simulink model "FW_formation_control_wind"  (R2023b)
settings: Solver=FixedStepAuto  StartTime=0.0  StopTime=70  FixedStep=0.001  RelTol=1e-3
undefined symbols (not defined in the file or in its folder): C, com, fc, hc, init, L, L2, lc, leader, tau, Va_max, Va_min
libraries: Fixed_Wing x3, simulink x1
(part 1 of 2)
settings Model: Creator=TigerWuu  LastModifiedBy=NCS
settings SolverCC: MaxConsecutiveMinStep=10  ZeroCrossAlgorithm=Adaptive  EnableFixedStepZeroCrossing=on
settings OptimizationCC: EnhancedBackFolding=on  PassReuseOutputArgsAs=Individual arguments  ZeroExternalMemoryAtStartup=off  ZeroInternalMemoryAtStartup=off  MaxStackSize=64  OptimizeBlockOrder=speed  DifferentSizesBufferReuse=on  OptimizationCustomize=off  EfficientTunableParamExpr=on
settings DebuggingCC: IgnoredZcDiagnostic=none  ParameterTunabilityLossMsg=error  UnconnectedInputMsg=warning  UnconnectedOutputMsg=warning  UnconnectedLineMsg=warning  UnderSpecifiedDimensionMsg=warning
settings HardwareCC: UseEmbeddedCoderFeatures=off
settings ModelReferenceCC: EnableRefExpFcnMdlSchedulingChecks=on
settings SFSimCC: MATLABDynamicMemAlloc=off
settings RTWCC: Description=Embedded Coder  SystemTargetFile=ert.tlc  HardwareBoard=Robot Operating System 2 (ROS 2)  TLCOptions="-aInlineSetEventsForThisBaseRateFcn=TLC_FALSE -aSuppressMultiTaskScheduler=TLC_FALSE  -aRateBasedStepFcn=0"  TemplateMakefile=ert_default_tmf  Toolchain=Colcon Tools  TargetLang=C++  DLArmComputeVersion=19.05
settings CodeAppCC: ForceParamTrailComments=on  IgnoreCustomStorageClasses=off  OperatorAnnotations=on  SimulinkDataObjDesc=on  SFDataObjDesc=on  InsertBlockDesc=on
settings ERTTargetCC: CodeInterfacePackaging=C++ class  SupportNonInlinedSFcns=on  RootIOFormat=Structure reference

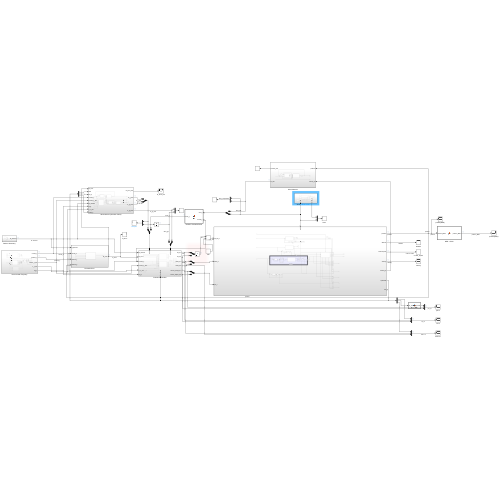
[thumbnail: Simulink's stored preview of the top-level diagram]
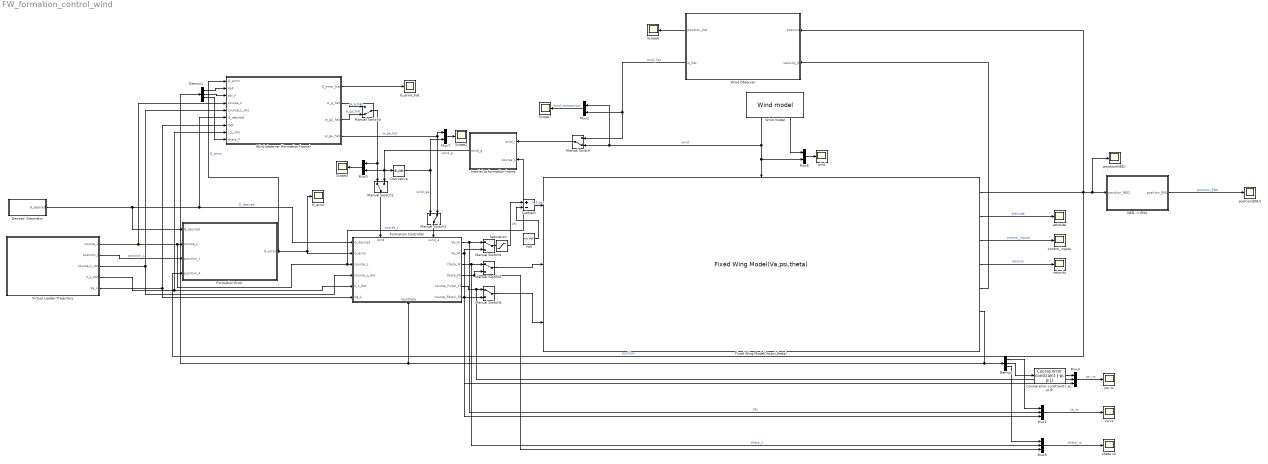
== system FW_formation_control_wind ==
  "Course error constraint [-pi, pi]1" : Fixed_Wing/Fixed Wing Model(Va,psi,theta)/Course error constraint [-pi, pi]1  SystemSampleTime=-1  VariantActivationTime=update diagram  AllowFlexibleInterface=on  Latency=0  AutoFrameSizeCalculation=off
      settings: SourceProductName=Fixed-Wing Model
  Demux : Demux  Outputs=3
  Demux1 : Demux  Outputs=3
  Derivative : Derivative
  Desired  Geometry : Subsystem
  Fixed Wing Model(Va,psi,theta) : Fixed_Wing/Fixed Wing Model(Va,psi,theta)  SystemSampleTime=-1  VariantActivationTime=update diagram  AllowFlexibleInterface=on  Latency=0  AutoFrameSizeCalculation=off
      link override Integrator: InitialCondition=init.psi0
      link override Integrator2: InitialCondition=init.psi0
      link override Ki_course: Gain=0
      settings: SourceProductName=Fixed-Wing Model  PortSchema="{\"entries\":[{\"content\":{\"sides\":[{\"content\":{\"connectorIds\":[\"In1\",\"In2\",\"In3\"]},\"type\":\"ConnectorPlacement.EquallySpacedRectSide\",\"uuid\":\"491080cc-ba33-4dca-9b37-922a1b131a7c\"},{\"content\":{\"connectorIds\":[\"Out1\",\"Out2\",\"Out3\",\"Out4\",\"Out5\",\"Out6\",\"Out7\"],\"side\":\"RIGHT\"},\"type\":\"ConnectorPlacement.EquallySpacedRectSide\",\"uuid\":\"e4e8ca81-264a-41b3-9d62-a2cb565f7b79\"},{\"content\":{\"connectorIds\":[\"In4\"],\"side\":\"TOP\"},\"type\":\"ConnectorPlacement.EquallySpacedRectSide\",\"uuid\":\"52444ebc-de17-4d3c-95e2-2270054ae63e\"},{\"content\":{\"side\":\"BOTTOM\"},\"type\":\"ConnectorPlacement.EquallySpacedRectSide\",\"uuid\":\"cd38afea-0687-422f-bcb3-a9854084c98f\"}]},\"type\":\"ConnectorPlacement.EquallySpacedConnector\",\"uuid\":\"020d1068-73e8-421c-b651-66bcdf43a07b\"}],\"packageUris\":[\"http://schema.mathworks.com/mf0/Connector/R2020b\"],\"version\":\"1.0\"}"
  Formation Controller : Subsystem
      settings: PortSchema="{\"entries\":[{\"content\":{\"sides\":[{\"content\":{\"connectorIds\":[\"In1\",\"In2\",\"In3\",\"In4\",\"In5\",\"In6\"]},\"type\":\"ConnectorPlacement.EquallySpacedRectSide\",\"uuid\":\"9c389f85-23f7-4ad0-9870-58a1e0934639\"},{\"content\":{\"connectorIds\":[\"Out1\",\"Out2\",\"Out3\",\"Out4\",\"Out5\",\"Out6\"],\"side\":\"RIGHT\"},\"type\":\"ConnectorPlacement.EquallySpacedRectSide\",\"uuid\":\"ce3247c4-1bae-44d3-b9da-13662f8788fa\"},{\"content\":{\"connectorIds\":[\"In7\",\"In8\"],\"side\":\"TOP\"},\"type\":\"ConnectorPlacement.EquallySpacedRectSide\",\"uuid\":\"1a627aed-9846-48b6-b280-b2fda66f57fb\"},{\"content\":{\"connectorIds\":[\"In9\"],\"side\":\"BOTTOM\"},\"type\":\"ConnectorPlacement.EquallySpacedRectSide\",\"uuid\":\"66985a5e-001d-400a-88a5-7872307471ad\"}]},\"type\":\"ConnectorPlacement.EquallySpacedConnector\",\"uuid\":\"4ccca4c3-7c97-47a5-8a1e-b96349422d36\"}],\"packageUris\":[\"http://schema.mathworks.com/mf0/Connector/R2020b\"],\"version\":\"1.0\"}"
  Formation Error : Subsystem
  G_error : Scope
  G_error_hat : Scope
  Inertial to formation frame : MATLAB Function  TreatAsAtomicUnit=on
  Manual Switch : ManualSwitch  CurrentSetting=0
  Manual Switch{1,4..6} (4 alike) : ManualSwitch
  Manual Switch2 : ManualSwitch  CurrentSetting=0
  Manual Switch3 : ManualSwitch  CurrentSetting=0
  Mux1 : Mux  Inputs=3
  Mux{2..3,6..7} (4 alike) : Mux  Inputs=2
  Mux4 : Mux  Inputs=3
  Mux5 : Mux  Inputs=3
  "NED -> ENU" : MATLAB Function  TreatAsAtomicUnit=on
  Saturation : Saturate  UpperLimit=Va_max  LowerLimit=Va_min
  Scope{2..3,6..7} (4 alike) : Scope
  Subtract : Sum  Inputs=+-
  Va0 : Constant  Value=init.Va0
  Virtual Leader Trajectory : Subsystem
  Wind Observer : Subsystem
  Wind model : Fixed_Wing/Wind model  SystemSampleTime=-1  VariantActivationTime=update diagram  AllowFlexibleInterface=on  Latency=0  AutoFrameSizeCalculation=off
      link override Steady wind /Gain: Gain=1
      link override Steady wind /Gain1: Gain=-2
      link override Steady wind /wd: Value=0
      link override Steady wind gust/Gain: Gain=0.2
      link override Steady wind gust/Gain1: Gain=0.2
      link override Steady wind gust/Gain2: Gain=1
      link override Steady wind gust/Gain3: Gain=-1
      link override Steady wind gust/Gain4: Gain=0.7
      settings: SourceProductName=Fixed-Wing Model  PortSchema="{\"entries\":[{\"content\":{\"sides\":[{\"content\":{},\"type\":\"ConnectorPlacement.EquallySpacedRectSide\",\"uuid\":\"19ef0eb7-c626-45ec-b76b-8668fc024824\"},{\"content\":{\"side\":\"RIGHT\"},\"type\":\"ConnectorPlacement.EquallySpacedRectSide\",\"uuid\":\"89e72569-ab94-4162-a6e2-b425ef08f724\"},{\"content\":{\"side\":\"TOP\"},\"type\":\"ConnectorPlacement.EquallySpacedRectSide\",\"uuid\":\"6d9409e9-6822-4cd9-902f-e5665cb68433\"},{\"content\":{\"connectorIds\":[\"Out1\",\"Out2\"],\"side\":\"BOTTOM\"},\"type\":\"ConnectorPlacement.EquallySpacedRectSide\",\"uuid\":\"39a83352-0924-44fa-be5d-94a7c28bbbf3\"}]},\"type\":\"ConnectorPlacement.EquallySpacedConnector\",\"uuid\":\"6cf6ae00-ef23-42a2-99b2-ca60e191fb03\"}],\"packageUris\":[\"http://schema.mathworks.com/mf0/Connector/R2020b\"],\"version\":\"1.0\"}"
  Wind observer (formation frame) : Subsystem
  attitude : Scope
  control_inputs : Scope
  position(ENU) : Scope
  position(NED) : Scope
  psi vs : Scope
  theta vs : Scope
  va vs : Scope
  velocity : Scope
  wind : Scope
  wires:
  Fixed Wing Model(Va,psi,theta)/1 -> position(NED)/1, "NED -> ENU"/1(position_NED), Formation Error/4(position_F), Wind Observer/1(position)  "position"
  Fixed Wing Model(Va,psi,theta)/3 -> control_inputs/1  "control_inputs"
  "NED -> ENU"/1(position_ENU) -> position(ENU)/1  "position_ENU"
  Virtual Leader Trajectory/2(position_L) -> Formation Error/3(position_L)  "position_L"
  Virtual Leader Trajectory/1(course_L) -> Wind observer (formation frame)/4(course_L), Inertial to formation frame/2(course_L), Formation Controller/3(course_L), Formation Error/2(course_L)  "course_L"
  Desired  Geometry/1(G_desired) -> Formation Error/1(G_desired), Wind observer (formation frame)/6(G_desired), Formation Controller/1(G_desired)  "G_desired"
  Virtual Leader Trajectory/3(course_L_dot) -> Formation Controller/4(course_L_dot), Wind observer (formation frame)/5(course_L_dot)
  Virtual Leader Trajectory/5(Vg_L) -> Formation Controller/6(Vg_L), Wind observer (formation frame)/7(VgL)
  Formation Error/1(G_error) -> Wind observer (formation frame)/1(G_error), G_error/1, Formation Controller/2(G_error)  "G_error"
  Wind model/1 -> Fixed Wing Model(Va,psi,theta)/4, Mux6/2, Mux2/1, Manual Switch/2  "wind"
  Formation Controller/5(course_Fc/psi_Fc) -> Mux4/2, Manual Switch6/1
  Fixed Wing Model(Va,psi,theta)/2 -> attitude/1  "attitude"
  Fixed Wing Model(Va,psi,theta)/4 -> velocity/1  "velocity"
  Subtract/1 -> Fixed Wing Model(Va,psi,theta)/1  "V_F_bar"
  Va0/1 -> Subtract/2
  Fixed Wing Model(Va,psi,theta)/5 -> Wind Observer/2(velocity_0)
  Wind Observer/1(position_hat) -> Scope6/1
  Mux2/1 -> Scope7/1  "wind_comparison"
  Wind Observer/2(w_hat) -> Manual Switch/1, Mux2/2  "wind_hat"
  Demux1/2 -> Wind observer (formation frame)/3(psi_F)
  Demux1/1 -> Wind observer (formation frame)/2(VaF)
  Fixed Wing Model(Va,psi,theta)/6 -> Demux/1, Demux1/1, Formation Controller/9(Vpsitheta)
  Wind observer (formation frame)/1(G_error_hat) -> G_error_hat/1
  Manual Switch/1 -> Inertial to formation frame/1(wind_i)
  Manual Switch1/1 -> Formation Controller/7(wind)
  Inertial to formation frame/1(wind_g) -> Mux3/2, Derivative/1, Manual Switch1/2  "wind_g"
  Mux3/1 -> Scope3/1
  Virtual Leader Trajectory/4(z_L_dot) -> Formation Controller/5(z_L_dot), Wind observer (formation frame)/8(z_L_dot)
  Saturation/1 -> Subtract/1  "VFc"
  Mux1/1 -> va vs/1  "va_vs"
  Mux4/1 -> psi vs/1  "psi_vs"
  Formation Controller/3(theta_Fc) -> Manual Switch5/1, Mux5/2  "theta_c"
  Mux5/1 -> theta vs/1  "theta_vs"
  Formation Controller/6(course_Fd/psi_Fd) -> Manual Switch6/2, Mux4/3
  Formation Controller/2(Va_Fd) -> Manual Switch4/2, Mux1/3
  Mux6/1 -> wind/1
  Wind model/2 -> Mux6/1
  Derivative/1 -> Manual Switch2/1, Mux7/2  "wind_ga"
  Mux7/1 -> Scope2/1
  Wind observer (formation frame)/4(w_ga_hat) -> Mux7/1, Manual Switch2/2  "w_ga_hat"
  Manual Switch2/1 -> Formation Controller/8(wind_a)
  Formation Controller/4(theta_Fd) -> Mux5/3, Manual Switch5/2
  Demux1/3 -> Wind observer (formation frame)/9(theta_F)
  Demux/1 -> Mux1/1
  Demux/2 -> "Course error constraint [-pi, pi]1"/1
  Demux/3 -> Mux5/1
  Wind observer (formation frame)/3(w_g2_hat) -> Manual Switch3/2  "w_g2_hat"
  Wind observer (formation frame)/2(w_g_hat) -> Manual Switch3/1  "w_g_hat"
  Manual Switch3/1 -> Manual Switch1/1, Mux3/1
  "Course error constraint [-pi, pi]1"/1 -> Mux4/1
  Formation Controller/1(Va_Fc) -> Mux1/2, Manual Switch4/1  "VFc"
  Manual Switch4/1 -> Saturation/1
  Manual Switch5/1 -> Fixed Wing Model(Va,psi,theta)/2
  Manual Switch6/1 -> Fixed Wing Model(Va,psi,theta)/3

== system FW_formation_control_wind/Desired  Geometry ==
  Mux : Mux  Inputs=3
  fc : Constant  Value=fc(2)
  hc : Constant  Value=hc(2)
  lc : Constant  Value=lc(2)
  G_desired : Outport
  wires:
  Mux/1 -> G_desired/1  "desired geometry"
  lc/1 -> Mux/1
  fc/1 -> Mux/2
  hc/1 -> Mux/3

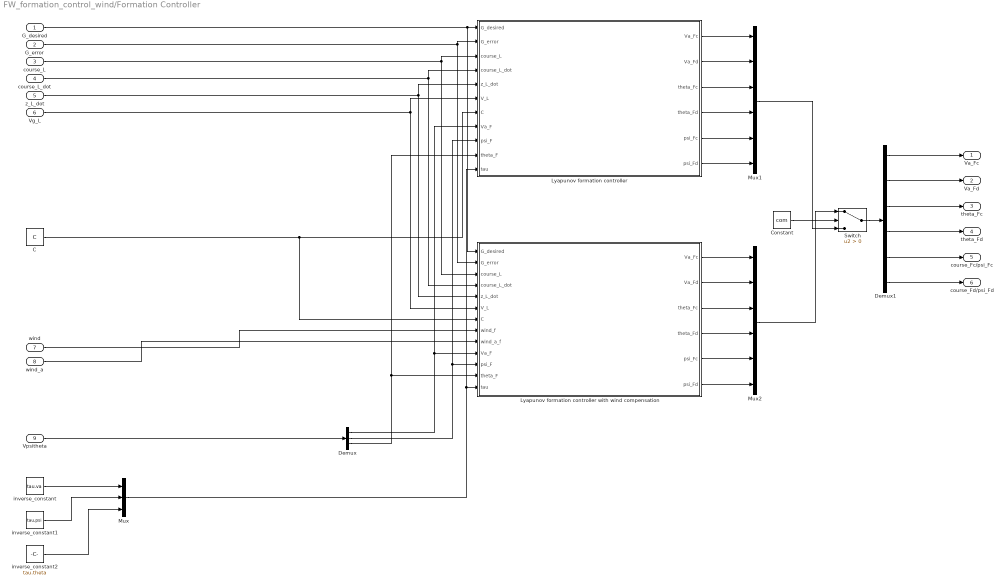
== system FW_formation_control_wind/Formation Controller ==
  G_desired : Inport
  G_error : Inport  Port=2
  course_L : Inport  Port=3
  course_L_dot : Inport  Port=4
  z_L_dot : Inport  Port=5
  Vg_L : Inport  Port=6
  wind : Inport  Port=7
  wind_a : Inport  Port=8
  Vpsitheta : Inport  Port=9
  C : Constant  Value=C
  Constant : Constant  Value=com
  Demux : Demux  Outputs=3
  Demux1 : Demux  Outputs=6
  Lyapunov formation controller : MATLAB Function  TreatAsAtomicUnit=on
  Lyapunov formation controller with wind compensation : MATLAB Function  TreatAsAtomicUnit=on
  Mux : Mux  Inputs=3
  Mux1 : Mux  Inputs=6
  Mux2 : Mux  Inputs=6
  Switch : Switch  Criteria=u2 > Threshold  SaturateOnIntegerOverflow=off  InputSameDT=off
  inverse_constant : Constant  Value=tau.va
  inverse_constant1 : Constant  Value=tau.psi
  inverse_constant2 : Constant  Value=tau.theta
  Va_Fc : Outport
  Va_Fd : Outport  Port=2
  theta_Fc : Outport  Port=3
  theta_Fd : Outport  Port=4
  course_Fc/psi_Fc : Outport  Port=5
  course_Fd/psi_Fd : Outport  Port=6
  wires:
  G_desired/1 -> Lyapunov formation controller with wind compensation/1(G_desired), Lyapunov formation controller/1(G_desired)
  course_L_dot/1 -> Lyapunov formation controller with wind compensation/4(course_L_dot), Lyapunov formation controller/4(course_L_dot)
  course_L/1 -> Lyapunov formation controller with wind compensation/3(course_L), Lyapunov formation controller/3(course_L)
  Vg_L/1 -> Lyapunov formation controller with wind compensation/6(V_L), Lyapunov formation controller/6(V_L)
  Demux1/1 -> Va_Fc/1
  wind/1 -> Lyapunov formation controller with wind compensation/8(wind_f)
  G_error/1 -> Lyapunov formation controller with wind compensation/2(G_error), Lyapunov formation controller/2(G_error)
  z_L_dot/1 -> Lyapunov formation controller with wind compensation/5(z_L_dot), Lyapunov formation controller/5(z_L_dot)
  Demux1/3 -> theta_Fc/1
  Vpsitheta/1 -> Demux/1
  Demux/1 -> Lyapunov formation controller/8(Va_F), Lyapunov formation controller with wind compensation/10(Va_F)
  Demux/2 -> Lyapunov formation controller/9(psi_F), Lyapunov formation controller with wind compensation/11(psi_F)
  Demux1/5 -> course_Fc/psi_Fc/1
  C/1 -> Lyapunov formation controller with wind compensation/7(C), Lyapunov formation controller/7(C)
  wind_a/1 -> Lyapunov formation controller with wind compensation/9(wind_a_f)
  Demux/3 -> Lyapunov formation controller with wind compensation/12(theta_F), Lyapunov formation controller/10(theta_F)
  inverse_constant1/1 -> Mux/2
  inverse_constant/1 -> Mux/1
  inverse_constant2/1 -> Mux/3
  Mux/1 -> Lyapunov formation controller/11(tau), Lyapunov formation controller with wind compensation/13(tau)
  Demux1/2 -> Va_Fd/1
  Demux1/4 -> theta_Fd/1
  Demux1/6 -> course_Fd/psi_Fd/1
  Lyapunov formation controller/1(Va_Fc) -> Mux1/1
  Lyapunov formation controller/2(Va_Fd) -> Mux1/2
  Lyapunov formation controller/3(theta_Fc) -> Mux1/3
  Lyapunov formation controller/4(theta_Fd) -> Mux1/4
  Lyapunov formation controller/5(psi_Fc) -> Mux1/5
  Lyapunov formation controller/6(psi_Fd) -> Mux1/6
  Lyapunov formation controller with wind compensation/1(Va_Fc) -> Mux2/1
  Lyapunov formation controller with wind compensation/2(Va_Fd) -> Mux2/2
  Lyapunov formation controller with wind compensation/3(theta_Fc) -> Mux2/3
  Lyapunov formation controller with wind compensation/4(theta_Fd) -> Mux2/4
  Lyapunov formation controller with wind compensation/6(psi_Fd) -> Mux2/6
  Lyapunov formation controller with wind compensation/5(psi_Fc) -> Mux2/5
  Constant/1 -> Switch/2
  Switch/1 -> Demux1/1
  Mux2/1 -> Switch/1
  Mux1/1 -> Switch/3

== system FW_formation_control_wind/Formation Error ==
  G_desired : Inport
  course_L : Inport  Port=2
  position_L : Inport  Port=3
  position_F : Inport  Port=4
  "Geometry error " : MATLAB Function  TreatAsAtomicUnit=on
  G_error : Outport
  wires:
  G_desired/1 -> "Geometry error "/1(G_desired)
  course_L/1 -> "Geometry error "/2(course_L)
  position_L/1 -> "Geometry error "/3(position_L)
  position_F/1 -> "Geometry error "/4(position_F)
  "Geometry error "/1(G_error) -> G_error/1

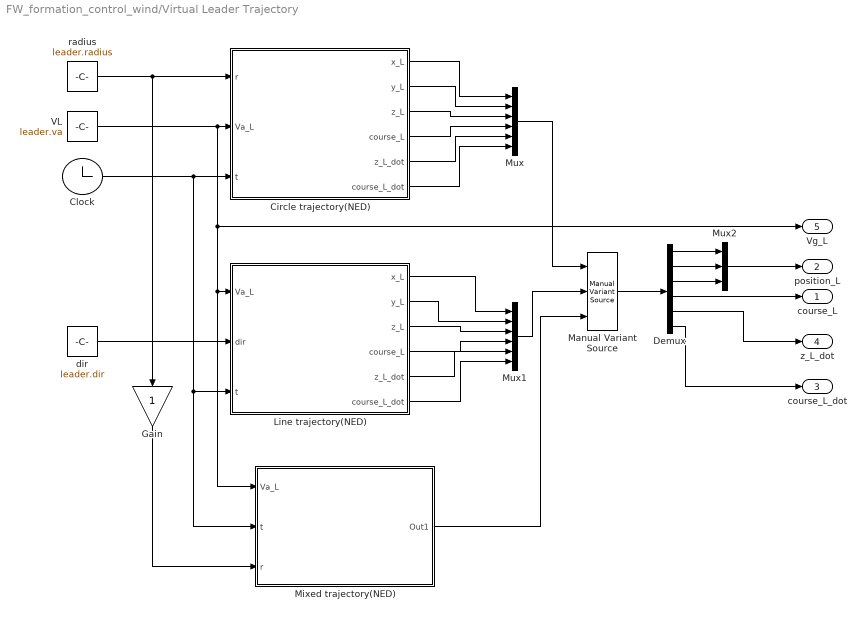
== system FW_formation_control_wind/Virtual Leader Trajectory ==
  Circle trajectory(NED) : MATLAB Function  TreatAsAtomicUnit=on
  Clock : Clock
  Demux : Demux  Outputs=6
  Gain : Gain
  Line trajectory(NED) : MATLAB Function  TreatAsAtomicUnit=on
  Manual Variant Source : simulink/Signal Routing/Manual Variant Source  NumChoices=3  LabelModeActiveChoice=V_2
  Mixed trajectory(NED) : Subsystem
  Mux : Mux  Inputs=6
  Mux1 : Mux  Inputs=6
  Mux2 : Mux  Inputs=3
  VL : Constant  Value=leader.va
  dir : Constant  Value=leader.dir
  radius : Constant  Value=leader.radius
  course_L : Outport
  position_L : Outport  Port=2
  course_L_dot : Outport  Port=3
  z_L_dot : Outport  Port=4
  Vg_L : Outport  Port=5
  wires:
  radius/1 -> Circle trajectory(NED)/1(r), Gain/1
  VL/1 -> Vg_L/1, Mixed trajectory(NED)/1(Va_L), Line trajectory(NED)/1(Va_L), Circle trajectory(NED)/2(Va_L)
  Clock/1 -> Mixed trajectory(NED)/2(t), Line trajectory(NED)/3(t), Circle trajectory(NED)/3(t)
  Mux/1 -> Manual Variant Source/1
  Circle trajectory(NED)/1(x_L) -> Mux/1
  Circle trajectory(NED)/2(y_L) -> Mux/2
  Circle trajectory(NED)/3(z_L) -> Mux/3
  Line trajectory(NED)/1(x_L) -> Mux1/1
  Line trajectory(NED)/2(y_L) -> Mux1/2
  Line trajectory(NED)/3(z_L) -> Mux1/3
  Line trajectory(NED)/4(course_L) -> Mux1/4
  Mux1/1 -> Manual Variant Source/2
  Manual Variant Source/1 -> Demux/1
  Demux/1 -> Mux2/1
  Demux/2 -> Mux2/2
  Demux/3 -> Mux2/3
  Mux2/1 -> position_L/1
  Circle trajectory(NED)/6(course_L_dot) -> Mux/6
  Line trajectory(NED)/6(course_L_dot) -> Mux1/6
  Line trajectory(NED)/5(z_L_dot) -> Mux1/5
  Demux/4 -> course_L/1
  Demux/5 -> z_L_dot/1
  Demux/6 -> course_L_dot/1
  Circle trajectory(NED)/4(course_L) -> Mux/4
  Circle trajectory(NED)/5(z_L_dot) -> Mux/5
  Gain/1 -> Mixed trajectory(NED)/3(r)
  Mixed trajectory(NED)/1(Out1) -> Manual Variant Source/3
  dir/1 -> Line trajectory(NED)/2(dir)

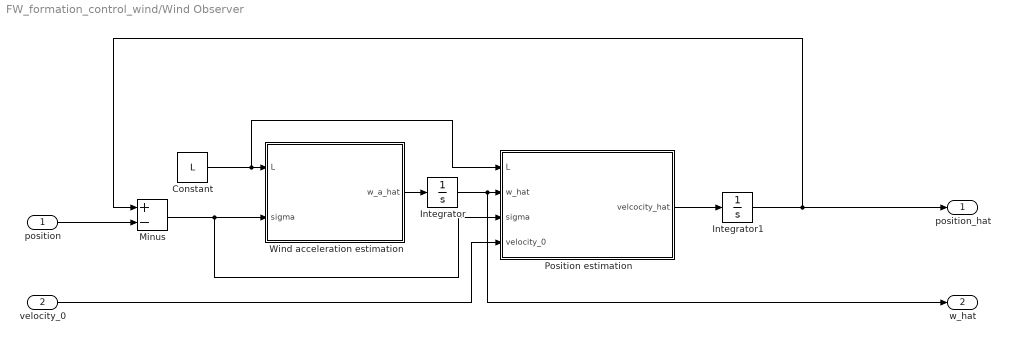
== system FW_formation_control_wind/Wind Observer ==
  position : Inport
  velocity_0 : Inport  Port=2
  Constant : Constant  Value=L
  Integrator : Integrator
  Integrator1 : Integrator
  Minus : Sum  Inputs=+-
  Position estimation : MATLAB Function  TreatAsAtomicUnit=on
  Wind acceleration estimation : MATLAB Function  TreatAsAtomicUnit=on
  position_hat : Outport
  w_hat : Outport  Port=2
  wires:
  Position estimation/1(velcocity_hat) -> Integrator1/1
  position/1 -> Minus/2
  Minus/1 -> Position estimation/3(sigma), Wind acceleration estimation/2(sigma)
  Wind acceleration estimation/1(w_a_hat) -> Integrator/1
  Constant/1 -> Position estimation/1(L), Wind acceleration estimation/1(L)
  Integrator1/1 -> Minus/1, position_hat/1
  Integrator/1 -> w_hat/1, Position estimation/2(w_hat)
  velocity_0/1 -> Position estimation/4(velocity_0)

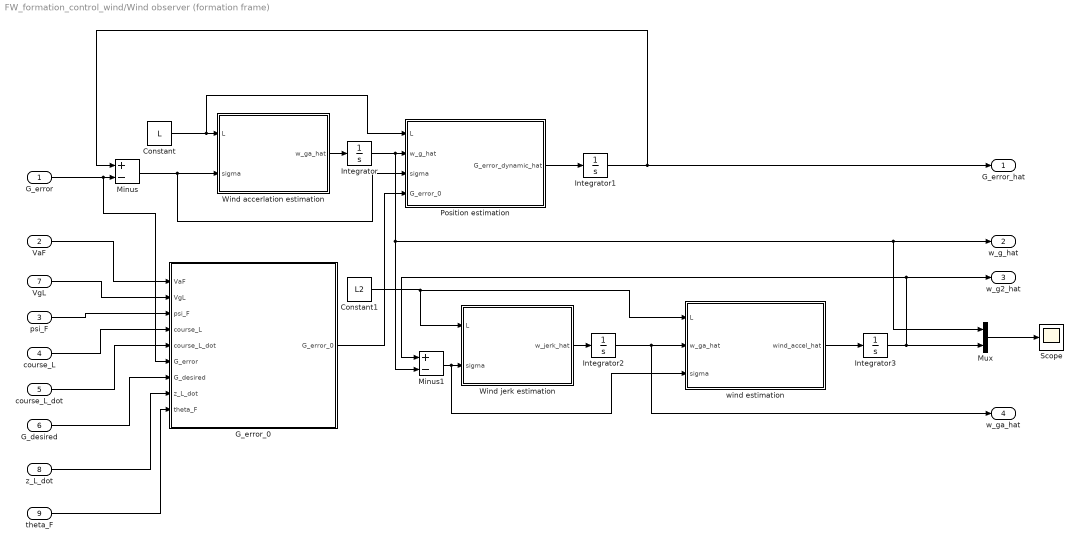
== system FW_formation_control_wind/Wind observer (formation frame) ==
  G_error : Inport
  VaF : Inport  Port=2
  psi_F : Inport  Port=3
  course_L : Inport  Port=4
  course_L_dot : Inport  Port=5
  G_desired : Inport  Port=6
  VgL : Inport  Port=7
  z_L_dot : Inport  Port=8
  theta_F : Inport  Port=9
  Constant : Constant  Value=L
  Constant1 : Constant  Value=L2
  G_error_0 : MATLAB Function  TreatAsAtomicUnit=on
  Integrator{,1..3} (4 alike) : Integrator
  Minus : Sum  Inputs=+-
  Minus1 : Sum  Inputs=+-
  Mux : Mux  Inputs=2
  Position estimation : MATLAB Function  TreatAsAtomicUnit=on
  Scope : Scope
  Wind accerlation estimation : MATLAB Function  TreatAsAtomicUnit=on
  Wind jerk estimation : MATLAB Function  TreatAsAtomicUnit=on
  wind estimation : MATLAB Function  TreatAsAtomicUnit=on
  G_error_hat : Outport
  w_g_hat : Outport  Port=2
  w_g2_hat : Outport  Port=3
  w_ga_hat : Outport  Port=4
  wires:
  Position estimation/1(G_error_dynamic_hat) -> Integrator1/1
  G_error/1 -> G_error_0/6(G_error), Minus/2
  Minus/1 -> Position estimation/3(sigma), Wind accerlation estimation/2(sigma)
  Wind accerlation estimation/1(w_ga_hat) -> Integrator/1
  Constant/1 -> Position estimation/1(L), Wind accerlation estimation/1(L)
  Integrator1/1 -> Minus/1, G_error_hat/1
  VaF/1 -> G_error_0/1(VaF)
  VgL/1 -> G_error_0/2(VgL)
  psi_F/1 -> G_error_0/3(psi_F)
  course_L/1 -> G_error_0/4(course_L)
  course_L_dot/1 -> G_error_0/5(course_L_dot)
  G_desired/1 -> G_error_0/7(G_desired)
  G_error_0/1(G_error_0) -> Position estimation/4(G_error_0)
  z_L_dot/1 -> G_error_0/8(z_L_dot)
  theta_F/1 -> G_error_0/9(theta_F)
  Minus1/1 -> wind estimation/3(sigma), Wind jerk estimation/2(sigma)
  Wind jerk estimation/1(w_jerk_hat) -> Integrator2/1
  Integrator2/1 -> w_ga_hat/1, wind estimation/2(w_ga_hat)
  wind estimation/1(wind_accel_hat) -> Integrator3/1
  Mux/1 -> Scope/1
  Constant1/1 -> Wind jerk estimation/1(L), wind estimation/1(L)
  Integrator3/1 -> Mux/2, Minus1/1, w_g2_hat/1
  Integrator/1 -> w_g_hat/1, Mux/1, Minus1/2, Position estimation/2(w_g_hat)

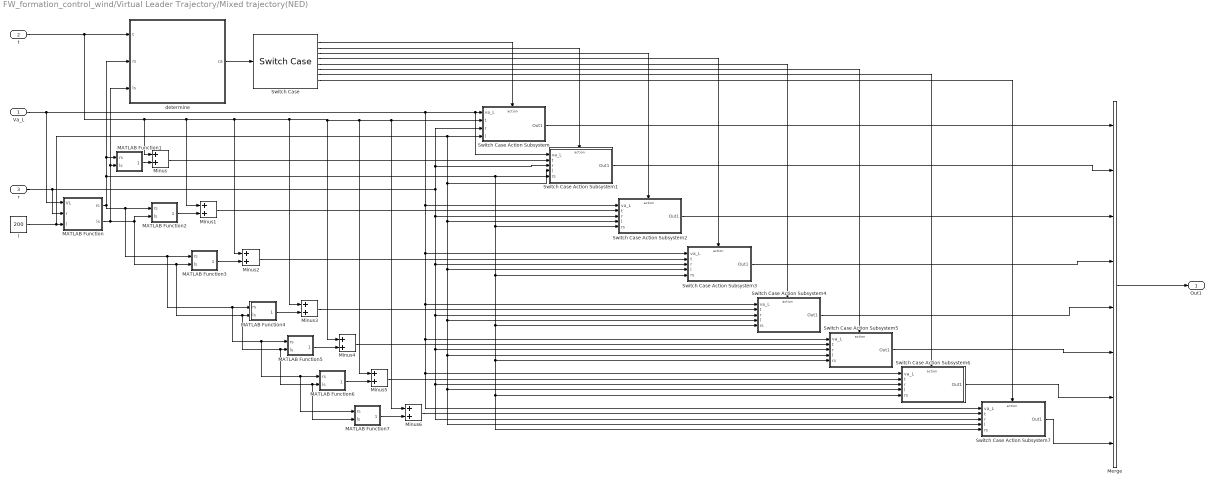
== system FW_formation_control_wind/Virtual Leader Trajectory/Mixed trajectory(NED) ==
  Va_L : Inport
  t : Inport  Port=2
  r : Inport  Port=3
  MATLAB Function : MATLAB Function  TreatAsAtomicUnit=on
  MATLAB Function1 : MATLAB Function  TreatAsAtomicUnit=on
  MATLAB Function2 : MATLAB Function  TreatAsAtomicUnit=on
  MATLAB Function3 : MATLAB Function  TreatAsAtomicUnit=on
  MATLAB Function4 : MATLAB Function  TreatAsAtomicUnit=on
  MATLAB Function5 : MATLAB Function  TreatAsAtomicUnit=on
  MATLAB Function6 : MATLAB Function  TreatAsAtomicUnit=on
  MATLAB Function7 : MATLAB Function  TreatAsAtomicUnit=on
  Merge : Merge  Inputs=8
  Minus{,1..6} (7 alike) : Sum
  Switch Case : SwitchCase  CaseConditions={1,2,3,4,5,6,7,8}  ShowDefaultCase=off
  Switch Case Action Subsystem : Subsystem  TreatAsAtomicUnit=on
  Switch Case Action Subsystem1 : Subsystem  TreatAsAtomicUnit=on
  Switch Case Action Subsystem2 : Subsystem  TreatAsAtomicUnit=on
  Switch Case Action Subsystem3 : Subsystem  TreatAsAtomicUnit=on
  Switch Case Action Subsystem4 : Subsystem  TreatAsAtomicUnit=on
  Switch Case Action Subsystem5 : Subsystem  TreatAsAtomicUnit=on
  Switch Case Action Subsystem6 : Subsystem  TreatAsAtomicUnit=on
  Switch Case Action Subsystem7 : Subsystem  TreatAsAtomicUnit=on
  determine : MATLAB Function  TreatAsAtomicUnit=on
  l : Constant  Value=200
  Out1 : Outport
  wires:
  determine/1(ca) -> Switch Case/1
  Switch Case/1 -> Switch Case Action Subsystem/Action
  MATLAB Function1/1(offset) -> Minus/2
  Switch Case/2 -> Switch Case Action Subsystem1/Action
  r/1 -> Switch Case Action Subsystem6/3(r), Switch Case Action Subsystem7/3(r), Switch Case Action Subsystem5/3(r), Switch Case Action Subsystem4/3(r), Switch Case Action Subsystem3/3(r), Switch Case Action Subsystem2/3(r), Switch Case Action Subsystem/3(r), Switch Case Action Subsystem1/3(r), MATLAB Function/2(r)
  MATLAB Function2/1(offset) -> Minus1/2
  Minus1/1 -> Switch Case Action Subsystem2/2(t)
  Switch Case/3 -> Switch Case Action Subsystem2/Action
  Switch Case/4 -> Switch Case Action Subsystem3/Action
  Minus/1 -> Switch Case Action Subsystem1/2(t)
  MATLAB Function3/1(offset) -> Minus2/2
  Minus2/1 -> Switch Case Action Subsystem3/2(t)
  Va_L/1 -> Switch Case Action Subsystem1/1(va_L), Switch Case Action Subsystem/1(va_L), Switch Case Action Subsystem4/1(va_L), Switch Case Action Subsystem5/1(va_L), Switch Case Action Subsystem6/1(va_L), Switch Case Action Subsystem7/1(va_L), Switch Case Action Subsystem3/1(va_L), Switch Case Action Subsystem2/1(va_L), MATLAB Function/1(VL)
  Minus3/1 -> Switch Case Action Subsystem4/2(t)
  Switch Case/5 -> Switch Case Action Subsystem4/Action
  MATLAB Function4/1(offset) -> Minus3/2
  Switch Case/6 -> Switch Case Action Subsystem5/Action
  MATLAB Function5/1(offset) -> Minus4/2
  Minus4/1 -> Switch Case Action Subsystem5/2(t)
  Switch Case/7 -> Switch Case Action Subsystem6/Action
  MATLAB Function6/1(offset) -> Minus5/2
  Minus5/1 -> Switch Case Action Subsystem6/2(t)
  Switch Case/8 -> Switch Case Action Subsystem7/Action
  t/1 -> Minus/1, Minus1/1, Minus2/1, Minus3/1, Minus4/1, Minus5/1, Minus6/1, Switch Case Action Subsystem/2(t), determine/1(t)
  Minus6/1 -> Switch Case Action Subsystem7/2(t)
  MATLAB Function7/1(offset) -> Minus6/2
  Switch Case Action Subsystem/1(Out1) -> Merge/1
  Switch Case Action Subsystem1/1(Out1) -> Merge/2
  Switch Case Action Subsystem2/1(Out1) -> Merge/3
  Switch Case Action Subsystem3/1(Out1) -> Merge/4
  Switch Case Action Subsystem4/1(Out1) -> Merge/5
  Switch Case Action Subsystem5/1(Out1) -> Merge/6
  Switch Case Action Subsystem6/1(Out1) -> Merge/7
  Switch Case Action Subsystem7/1(Out1) -> Merge/8
  Merge/1 -> Out1/1
  l/1 -> Switch Case Action Subsystem/4(l), Switch Case Action Subsystem5/4(l), Switch Case Action Subsystem6/4(l), Switch Case Action Subsystem7/4(l), Switch Case Action Subsystem4/4(l), Switch Case Action Subsystem3/4(l), Switch Case Action Subsystem2/4(l), Switch Case Action Subsystem1/4(l), MATLAB Function/3(l)
  MATLAB Function/1(rs) -> MATLAB Function7/1(rs), MATLAB Function6/1(rs), MATLAB Function5/1(rs), MATLAB Function4/1(rs), MATLAB Function3/1(rs), MATLAB Function2/1(rs), MATLAB Function1/1(rs), determine/2(rs), Switch Case Action Subsystem4/5(rs), Switch Case Action Subsystem5/5(rs), Switch Case Action Subsystem6/5(rs), Switch Case Action Subsystem7/5(rs), Switch Case Action Subsystem3/5(rs), Switch Case Action Subsystem2/5(rs), Switch Case Action Subsystem1/5(rs)
  MATLAB Function/2(ls) -> MATLAB Function7/2(ls), MATLAB Function6/2(ls), MATLAB Function5/2(ls), MATLAB Function4/2(ls), MATLAB Function3/2(ls), MATLAB Function2/2(ls), MATLAB Function1/2(ls), determine/3(ls)

== system FW_formation_control_wind/Virtual Leader Trajectory/Mixed trajectory(NED)/Switch Case Action Subsystem ==
  va_L : Inport
  t : Inport  Port=2
  r : Inport  Port=3
  l : Inport  Port=4
  Action Port : ActionPort  ActionPortLabel=case [ 1 ]:
  Line trajectory(NED) : MATLAB Function  TreatAsAtomicUnit=on
  Mux : Mux  Inputs=6
  Out1 : Outport
  wires:
  t/1 -> Line trajectory(NED)/2(t)
  va_L/1 -> Line trajectory(NED)/1(Va_L)
  Line trajectory(NED)/6(course_L_dot) -> Mux/6
  Line trajectory(NED)/5(z_L_dot) -> Mux/5
  Line trajectory(NED)/4(course_L) -> Mux/4
  Line trajectory(NED)/3(z_L) -> Mux/3
  Line trajectory(NED)/2(y_L) -> Mux/2
  Line trajectory(NED)/1(x_L) -> Mux/1
  Mux/1 -> Out1/1
  r/1 -> Line trajectory(NED)/3(r)
  l/1 -> Line trajectory(NED)/4(l)

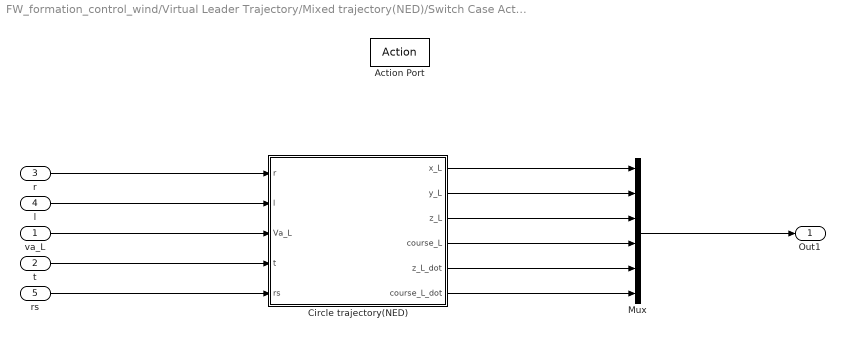
== system FW_formation_control_wind/Virtual Leader Trajectory/Mixed trajectory(NED)/Switch Case Action Subsystem1 ==
  va_L : Inport
  t : Inport  Port=2
  r : Inport  Port=3
  l : Inport  Port=4
  rs : Inport  Port=5
  Action Port : ActionPort  ActionPortLabel=case [ 2 ]:
  Circle trajectory(NED) : MATLAB Function  TreatAsAtomicUnit=on
  Mux : Mux  Inputs=6
  Out1 : Outport
  wires:
  t/1 -> Circle trajectory(NED)/4(t)
  va_L/1 -> Circle trajectory(NED)/3(Va_L)
  Circle trajectory(NED)/6(course_L_dot) -> Mux/6
  Circle trajectory(NED)/5(z_L_dot) -> Mux/5
  Circle trajectory(NED)/4(course_L) -> Mux/4
  Circle trajectory(NED)/3(z_L) -> Mux/3
  Circle trajectory(NED)/2(y_L) -> Mux/2
  Circle trajectory(NED)/1(x_L) -> Mux/1
  Mux/1 -> Out1/1
  r/1 -> Circle trajectory(NED)/1(r)
  l/1 -> Circle trajectory(NED)/2(l)
  rs/1 -> Circle trajectory(NED)/5(rs)

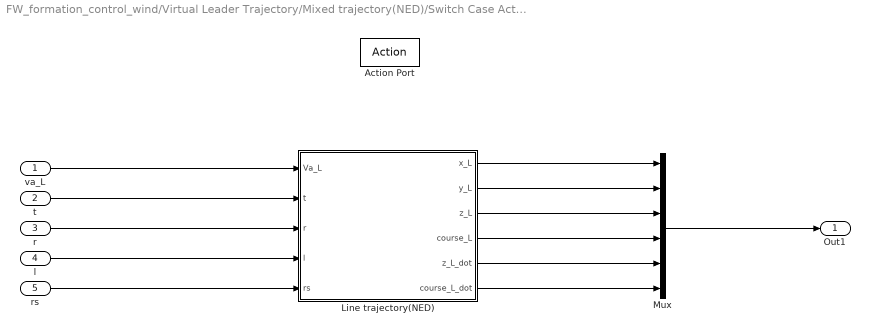
== system FW_formation_control_wind/Virtual Leader Trajectory/Mixed trajectory(NED)/Switch Case Action Subsystem2 ==
  va_L : Inport
  t : Inport  Port=2
  r : Inport  Port=3
  l : Inport  Port=4
  rs : Inport  Port=5
  Action Port : ActionPort  ActionPortLabel=case [ 3 ]:
  Line trajectory(NED) : MATLAB Function  TreatAsAtomicUnit=on
  Mux : Mux  Inputs=6
  Out1 : Outport
  wires:
  t/1 -> Line trajectory(NED)/2(t)
  va_L/1 -> Line trajectory(NED)/1(Va_L)
  Line trajectory(NED)/6(course_L_dot) -> Mux/6
  Line trajectory(NED)/5(z_L_dot) -> Mux/5
  Line trajectory(NED)/4(course_L) -> Mux/4
  Line trajectory(NED)/3(z_L) -> Mux/3
  Line trajectory(NED)/2(y_L) -> Mux/2
  Line trajectory(NED)/1(x_L) -> Mux/1
  Mux/1 -> Out1/1
  rs/1 -> Line trajectory(NED)/5(rs)
  l/1 -> Line trajectory(NED)/4(l)
  r/1 -> Line trajectory(NED)/3(r)

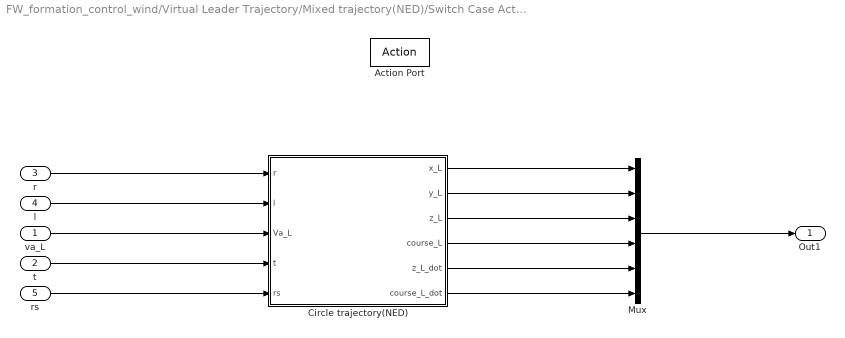
== system FW_formation_control_wind/Virtual Leader Trajectory/Mixed trajectory(NED)/Switch Case Action Subsystem3 ==
  va_L : Inport
  t : Inport  Port=2
  r : Inport  Port=3
  l : Inport  Port=4
  rs : Inport  Port=5
  Action Port : ActionPort  ActionPortLabel=case [ 4 ]:
  Circle trajectory(NED) : MATLAB Function  TreatAsAtomicUnit=on
  Mux : Mux  Inputs=6
  Out1 : Outport
  wires:
  t/1 -> Circle trajectory(NED)/4(t)
  va_L/1 -> Circle trajectory(NED)/3(Va_L)
  Circle trajectory(NED)/6(course_L_dot) -> Mux/6
  Circle trajectory(NED)/5(z_L_dot) -> Mux/5
  Circle trajectory(NED)/4(course_L) -> Mux/4
  Circle trajectory(NED)/3(z_L) -> Mux/3
  Circle trajectory(NED)/2(y_L) -> Mux/2
  Circle trajectory(NED)/1(x_L) -> Mux/1
  Mux/1 -> Out1/1
  r/1 -> Circle trajectory(NED)/1(r)
  rs/1 -> Circle trajectory(NED)/5(rs)
  l/1 -> Circle trajectory(NED)/2(l)

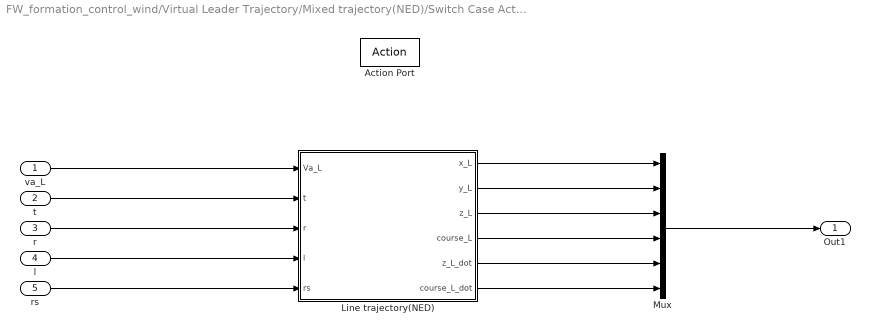
== system FW_formation_control_wind/Virtual Leader Trajectory/Mixed trajectory(NED)/Switch Case Action Subsystem4 ==
  va_L : Inport
  t : Inport  Port=2
  r : Inport  Port=3
  l : Inport  Port=4
  rs : Inport  Port=5
  Action Port : ActionPort  ActionPortLabel=case [ 5 ]:
  Line trajectory(NED) : MATLAB Function  TreatAsAtomicUnit=on
  Mux : Mux  Inputs=6
  Out1 : Outport
  wires:
  t/1 -> Line trajectory(NED)/2(t)
  va_L/1 -> Line trajectory(NED)/1(Va_L)
  Line trajectory(NED)/6(course_L_dot) -> Mux/6
  Line trajectory(NED)/5(z_L_dot) -> Mux/5
  Line trajectory(NED)/4(course_L) -> Mux/4
  Line trajectory(NED)/3(z_L) -> Mux/3
  Line trajectory(NED)/2(y_L) -> Mux/2
  Line trajectory(NED)/1(x_L) -> Mux/1
  Mux/1 -> Out1/1
  r/1 -> Line trajectory(NED)/3(r)
  l/1 -> Line trajectory(NED)/4(l)
  rs/1 -> Line trajectory(NED)/5(rs)

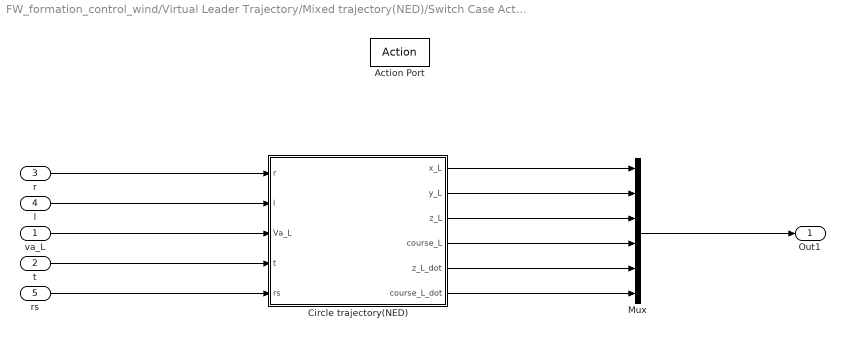
== system FW_formation_control_wind/Virtual Leader Trajectory/Mixed trajectory(NED)/Switch Case Action Subsystem5 ==
  va_L : Inport
  t : Inport  Port=2
  r : Inport  Port=3
  l : Inport  Port=4
  rs : Inport  Port=5
  Action Port : ActionPort  ActionPortLabel=case [ 6 ]:
  Circle trajectory(NED) : MATLAB Function  TreatAsAtomicUnit=on
  Mux : Mux  Inputs=6
  Out1 : Outport
  wires:
  t/1 -> Circle trajectory(NED)/4(t)
  va_L/1 -> Circle trajectory(NED)/3(Va_L)
  Circle trajectory(NED)/6(course_L_dot) -> Mux/6
  Circle trajectory(NED)/5(z_L_dot) -> Mux/5
  Circle trajectory(NED)/4(course_L) -> Mux/4
  Circle trajectory(NED)/3(z_L) -> Mux/3
  Circle trajectory(NED)/2(y_L) -> Mux/2
  Circle trajectory(NED)/1(x_L) -> Mux/1
  Mux/1 -> Out1/1
  r/1 -> Circle trajectory(NED)/1(r)
  rs/1 -> Circle trajectory(NED)/5(rs)
  l/1 -> Circle trajectory(NED)/2(l)

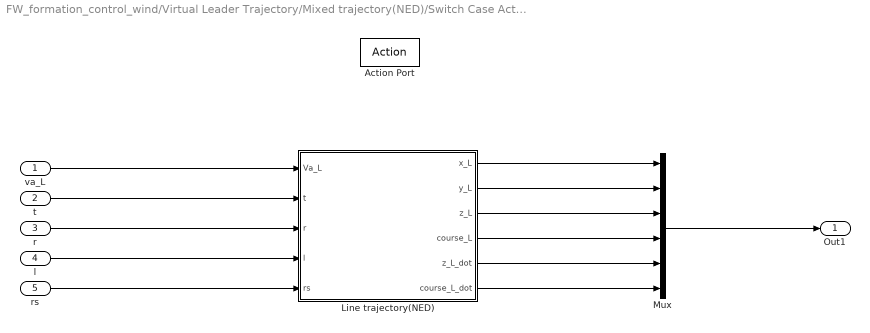
== system FW_formation_control_wind/Virtual Leader Trajectory/Mixed trajectory(NED)/Switch Case Action Subsystem6 ==
  va_L : Inport
  t : Inport  Port=2
  r : Inport  Port=3
  l : Inport  Port=4
  rs : Inport  Port=5
  Action Port : ActionPort  ActionPortLabel=case [ 7 ]:
  Line trajectory(NED) : MATLAB Function  TreatAsAtomicUnit=on
  Mux : Mux  Inputs=6
  Out1 : Outport
  wires:
  t/1 -> Line trajectory(NED)/2(t)
  va_L/1 -> Line trajectory(NED)/1(Va_L)
  Line trajectory(NED)/6(course_L_dot) -> Mux/6
  Line trajectory(NED)/5(z_L_dot) -> Mux/5
  Line trajectory(NED)/4(course_L) -> Mux/4
  Line trajectory(NED)/3(z_L) -> Mux/3
  Line trajectory(NED)/2(y_L) -> Mux/2
  Line trajectory(NED)/1(x_L) -> Mux/1
  Mux/1 -> Out1/1
  r/1 -> Line trajectory(NED)/3(r)
  l/1 -> Line trajectory(NED)/4(l)
  rs/1 -> Line trajectory(NED)/5(rs)

== system FW_formation_control_wind/Virtual Leader Trajectory/Mixed trajectory(NED)/Switch Case Action Subsystem7 ==
  va_L : Inport
  t : Inport  Port=2
  r : Inport  Port=3
  l : Inport  Port=4
  rs : Inport  Port=5
  Action Port : ActionPort  ActionPortLabel=case [ 8 ]:
  Circle trajectory(NED) : MATLAB Function  TreatAsAtomicUnit=on
  Mux : Mux  Inputs=6
  Out1 : Outport
  wires:
  t/1 -> Circle trajectory(NED)/4(t)
  va_L/1 -> Circle trajectory(NED)/3(Va_L)
  Circle trajectory(NED)/6(course_L_dot) -> Mux/6
  Circle trajectory(NED)/5(z_L_dot) -> Mux/5
  Circle trajectory(NED)/4(course_L) -> Mux/4
  Circle trajectory(NED)/3(z_L) -> Mux/3
  Circle trajectory(NED)/2(y_L) -> Mux/2
  Circle trajectory(NED)/1(x_L) -> Mux/1
  Mux/1 -> Out1/1
  r/1 -> Circle trajectory(NED)/1(r)
  l/1 -> Circle trajectory(NED)/2(l)
  rs/1 -> Circle trajectory(NED)/5(rs)

== matlab function FW_formation_control_wind/Wind Observer/Wind acceleration estimation ==
  data: L input; sigma input; w_a_hat output
function w_a_hat = WAEstimation(L, sigma)
    lamda0 = 1.1*L;
    w_a_hat = -lamda0*sign(sigma); 
end

== matlab function FW_formation_control_wind/Wind Observer/Position estimation ==
  data: L input; w_hat input; sigma input; velcocity_hat output; velocity_0 input
function velcocity_hat = velocityEstimation(L, w_hat, sigma, velocity_0)
    lambda1 = 1.5*L^(1/2);
    velcocity_hat = velocity_0 - lambda1*(abs(sigma).^(1/2).*sign(sigma))+ w_hat;
end

== matlab function FW_formation_control_wind/Inertial to formation frame ==
  data: wind_i input; wind_g output; course_L input
function wind_g = fcn(wind_i, course_L)
    phi_L = 0; % assume zero first
    theta_L = 0; % assume zero first
    R_r = [1, 0     , 0     ;   
           0, cos(phi_L), -sin(phi_L);
           0, sin(phi_L),  cos(phi_L)];
    R_p = [cos(theta_L), 0, sin(theta_L);
             0     , 1, 0     ;
            -sin(theta_L), 0, cos(theta_L)];
    R_y = [cos(course_L), -sin(course_L), 0;
           sin(course_L),  cos(course_L), 0;
           0     ,  0     , 1];
    % inertial to body
    R = R_y*R_p*R_r;
    wind_b = transpose(R)* wind_i;
    % body to formation frame
    wind_g = [wind_b(2);-wind_b(1); wind_b(3)]; % wl, wf, wh
end

== matlab function FW_formation_control_wind/Formation Controller/Lyapunov formation controller with wind compensation ==
  data: Va_Fc output size=1; G_desired input; G_error input; course_L input; course_L_dot input; z_L_dot input; V_L input; Va_Fd output size=1; theta_Fc output size=1; theta_Fd output size=1; psi_Fc output size=1; psi_Fd output size=1; C input; wind_f input; wind_a_f input; Va_F input; psi_F input; theta_F input; tau input
function [Va_Fc, Va_Fd,theta_Fc , theta_Fd, psi_Fc , psi_Fd] = lyapunov_formation(G_desired, G_error, course_L, course_L_dot, z_L_dot, V_L, C, wind_f, wind_a_f, Va_F, psi_F, theta_F, tau)
    lc = G_desired(1);
    fc = G_desired(2);
    hc = G_desired(3);
    le = G_error(1);
    fe = G_error(2);
    he = G_error(3);
    wl = wind_f(1);
    wf = wind_f(2);
    wh = wind_f(3);
    wl_dot = wind_a_f(1);
    wf_dot = wind_a_f(2);
    wh_dot = wind_a_f(3);
    % wl_dot = 0;
    % wf_dot = 0;
    % wh_dot = 0;
    
    c1 = C(1);
    c2 = C(2);
    c3 = C(3);
    c4 = C(4);
    c5 = C(5);
    c6 = C(6);


    Va_Fd = sqrt((c1*le+course_L_dot*fc+wl)^2+(c2*fe-course_L_dot*lc+V_L+wf)^2);
    psi_Fd = atan2(-c1*le-course_L_dot*fc-wl, c2*fe-course_L_dot*lc+V_L+wf)+course_L;
    while psi_Fd < -pi
        psi_Fd = psi_Fd + 2*pi;
    end
    while psi_Fd > pi
        psi_Fd = psi_Fd - 2*pi;
    end 
    % derive command
    V_L_dot = 0;
    le_dot = Va_F*sin(psi_F-course_L)+course_L_dot*(fe+fc)+wl;
    fe_dot = V_L-Va_F*cos(psi_F-course_L)-course_L_dot*(le+lc)+wf;
    he_dot = -z_L_dot-Va_F*sin(theta_F)+wh;

    a = -c1*le-course_L_dot*fc-wl;
    a_dot = -c1*le_dot-wl_dot;
    b = c2*fe-course_L_dot*lc+V_L+wf;
    b_dot = c2*fe_dot+V_L_dot+wf_dot;
    c = c3*he-z_L_dot+wh;
    c_dot = c3*he_dot+wh_dot;
    % ensure that the value in asin funtion fall between [-1,1]
    if c > Va_Fd
        c = Va_Fd;
    elseif c < -Va_Fd
        c = -Va_Fd;
    end

    theta_Fd = asin(c/Va_Fd);

   
    psie = psi_F-psi_Fd;
    Va_Fe = Va_F-Va_Fd;
    theta_Fe = theta_F-theta_Fd;

    while psie < -pi
        psie = psie + 2*pi;
    end
    while psie > pi
        psie = psie - 2*pi;
    end

    alpha = tau(1);
    beta = tau(2);
    gamma = tau(3);

    
    Va_Fc = 1/alpha*((a_dot*a+b*b_dot)/sqrt(a^2+b^2)-c4*Va_Fe)+Va_F;
    psi_Fc = 1/beta*((a_dot*b-a*b_dot)/(a^2+b^2)+course_L_dot-c5*psie)+psi_F;
    theta_Fc = 1/gamma*((c_dot*Va_Fd-c*((a_dot*a+b*b_dot)/sqrt(a^2+b^2)))/(Va_Fd*sqrt(Va_Fd^2-c^2))-c6*theta_Fe)+theta_F;
    
    while psi_Fc < -pi
        psi_Fc = psi_Fc + 2*pi;
    end
    while psi_Fc > pi
        psi_Fc = psi_Fc - 2*pi;
    end

end

== matlab function FW_formation_control_wind/Wind observer (formation frame)/Wind accerlation estimation ==
  data: L input; sigma input; w_ga_hat output
function w_ga_hat = WAEstimation(L, sigma)
    lamda0 = 1.1*L;
    w_ga_hat = -lamda0*sign(sigma); 
end

== matlab function FW_formation_control_wind/Wind observer (formation frame)/G_error_0 ==
  data: VaF input; VgL input; psi_F input; course_L input; course_L_dot input; G_error input; G_desired input; G_error_0 output; z_L_dot input; theta_F input
function G_error_0 = fcn(VaF,VgL, psi_F, course_L, course_L_dot, G_error, G_desired, z_L_dot, theta_F)
    G_error_0 = zeros(3,1);
    le = G_error(1);
    fe = G_error(2);
    lc = G_desired(1);
    fc = G_desired(2);
    G_error_1 = VaF*sin(psi_F-course_L)+course_L_dot*(fe+fc);
    G_error_2 = VgL-VaF*cos(psi_F-course_L)-course_L_dot*(le+lc);
    G_error_3 = -z_L_dot-VaF*sin(theta_F);
    G_error_0 = [G_error_1;G_error_2;G_error_3]; % error_3 will slow down the simulation
end

== matlab function FW_formation_control_wind/Virtual Leader Trajectory/Circle trajectory(NED) ==
  data: x_L output; y_L output; z_L output; course_L output; z_L_dot output; course_L_dot output; r input; Va_L input; t input
  function [x_L, y_L, z_L, course_L, z_L_dot, course_L_dot] = trajectory_generation(r,Va_L, t)
    climbing_rate = -1; % 3D
    Va_Lp = sqrt(Va_L^2-climbing_rate^2);
    omega = Va_Lp/r; % rad/s
    x_L = r*cos(omega*t);
    y_L = r*sin(omega*t);
    z_L = -90+climbing_rate*t; % 3D
    % z_L = -90+10*sin(3*omega*t); % 3D
    % z_L = -90; %2D
    
    x_L_dot = -r*omega*sin(omega*t);
    y_L_dot = r*omega*cos(omega*t);
    z_L_dot = climbing_rate; % 3D
    % z_L_dot = 30*cos(3*omega*t); % 3D
    % z_L_dot = 0; % 2D
    x_L_dotdot = -r*omega^2*cos(omega*t);
    y_L_dotdot = -r*omega^2*sin(omega*t);
    course_L = atan2(y_L_dot,x_L_dot);
    course_L_dot = (y_L_dotdot*x_L_dot-x_L_dotdot*y_L_dot)/(x_L_dot^2+y_L_dot^2);
end

== matlab function FW_formation_control_wind/Virtual Leader Trajectory/Line trajectory(NED) ==
  data: Va_L input; dir input; x_L output; y_L output; z_L output; course_L output; z_L_dot output; course_L_dot output; t input
function [x_L, y_L, z_L, course_L, z_L_dot, course_L_dot] = trajectory_generation(Va_L,dir, t)
    climbing_rate = -1; % 3D
    Va_Lp = sqrt(Va_L^2-climbing_rate^2);
    x_L = Va_Lp*t*cos(dir);    
    y_L = Va_Lp*t*sin(dir);
    % z_L = -90;
    z_L = -90+climbing_rate*t; % 3D
    x_L_dot = Va_Lp*cos(dir);
    y_L_dot = Va_Lp*sin(dir);
    % z_L_dot = 0;
    z_L_dot = climbing_rate; % 3D
    course_L = atan2(y_L_dot,x_L_dot);
    course_L_dot = 0;
end

== matlab function FW_formation_control_wind/Virtual Leader Trajectory/Mixed trajectory(NED)/Switch Case Action Subsystem2/Line trajectory(NED) ==
  data: x_L output; y_L output; z_L output; course_L output; z_L_dot output; course_L_dot output; Va_L input; t input; r input; l input; rs input
function [x_L, y_L, z_L, course_L, z_L_dot, course_L_dot] = trajectory_generation(Va_L, t,r,l, rs)
    climbing_rate = 0; % 3D
    Va_Lp = sqrt(Va_L^2-climbing_rate^2);
    x_L = l/2+Va_Lp*t*sin(3/2*pi);    
    y_L = -l/2-r;
    % z_L = -90;
    z_L = -90-2*rs; % 3D
    x_L_dot = Va_Lp*sin(3/2*pi);
    y_L_dot = 0;
    % z_L_dot = 0;
    z_L_dot = climbing_rate; % 3D
    course_L = atan2(y_L_dot,x_L_dot);
    course_L_dot = 0;
end

== matlab function FW_formation_control_wind/Virtual Leader Trajectory/Mixed trajectory(NED)/Switch Case Action Subsystem1/Circle trajectory(NED) ==
  data: x_L output; y_L output; z_L output; course_L output; z_L_dot output; course_L_dot output; r input; l input; Va_L input; t input; rs input
  function [x_L, y_L, z_L, course_L, z_L_dot, course_L_dot] = trajectory_generation(r,l,Va_L, t, rs)
    t1 = t - rs;
    climbing_rate = -2; % 3D
    Va_Lp = sqrt(Va_L^2-climbing_rate^2);
    omega = Va_Lp/r; % rad/s
    x_L = l/2+r*sin(omega*t);
    y_L = -l/2+r*cos(omega*t);
    z_L = -90+climbing_rate*t1; % 3D
    % z_L = -90+10*sin(3*omega*t); % 3D
    % z_L = -90; %2D
    
    x_L_dot = r*omega*cos(omega*t);
    y_L_dot = -r*omega*sin(omega*t);
    z_L_dot = climbing_rate; % 3D
    % z_L_dot = 30*cos(3*omega*t); % 3D
    % z_L_dot = 0; % 2D
    y_L_dotdot = -r*omega^2*cos(omega*t);
    x_L_dotdot = -r*omega^2*sin(omega*t);
    course_L = atan2(y_L_dot,x_L_dot);
    course_L_dot = (y_L_dotdot*x_L_dot-x_L_dotdot*y_L_dot)/(x_L_dot^2+y_L_dot^2);
end

== matlab function FW_formation_control_wind/Virtual Leader Trajectory/Mixed trajectory(NED)/Switch Case Action Subsystem3/Circle trajectory(NED) ==
  data: x_L output; y_L output; z_L output; course_L output; z_L_dot output; course_L_dot output; r input; l input; Va_L input; t input; rs input
  function [x_L, y_L, z_L, course_L, z_L_dot, course_L_dot] = trajectory_generation(r,l,Va_L, t, rs)
    t1 = t - 2*rs;
    climbing_rate = 2; % 3D
    Va_Lp = sqrt(Va_L^2-climbing_rate^2);
    omega = Va_Lp/r; % rad/s
    x_L = -l/2+r*sin(omega*t);
    y_L = -l/2+r*cos(omega*t);
    z_L = -90-2*rs+climbing_rate*t1; % 3D
    % z_L = -90+10*sin(3*omega*t); % 3D
    % z_L = -90; %2D
    
    x_L_dot = r*omega*cos(omega*t);
    y_L_dot = -r*omega*sin(omega*t);
    z_L_dot = climbing_rate; % 3D
    % z_L_dot = 30*cos(3*omega*t); % 3D
    % z_L_dot = 0; % 2D

    x_L_dotdot = -r*omega^2*sin(omega*t);
    y_L_dotdot = -r*omega^2*cos(omega*t);
    course_L = atan2(y_L_dot,x_L_dot);
    course_L_dot = (y_L_dotdot*x_L_dot-x_L_dotdot*y_L_dot)/(x_L_dot^2+y_L_dot^2);
end

== matlab function FW_formation_control_wind/Virtual Leader Trajectory/Mixed trajectory(NED)/Switch Case Action Subsystem4/Line trajectory(NED) ==
  data: x_L output; y_L output; z_L output; course_L output; z_L_dot output; course_L_dot output; Va_L input; t input; r input; l input; rs input
function [x_L, y_L, z_L, course_L, z_L_dot, course_L_dot] = trajectory_generation(Va_L, t,r,l, rs)
    climbing_rate = 0; % 3D
    Va_Lp = sqrt(Va_L^2-climbing_rate^2);
    x_L = -l/2-r;    
    y_L = -l/2+Va_Lp*t*cos(0);
    % z_L = -90;
    z_L = -90; % 3D

    x_L_dot = 0;
    y_L_dot = Va_Lp*cos(0);
    % z_L_dot = 0;
    z_L_dot = climbing_rate; % 3D
    course_L = atan2(y_L_dot,x_L_dot);
    course_L_dot = 0;
end

== matlab function FW_formation_control_wind/Virtual Leader Trajectory/Mixed trajectory(NED)/Switch Case Action Subsystem5/Circle trajectory(NED) ==
  data: x_L output; y_L output; z_L output; course_L output; z_L_dot output; course_L_dot output; r input; l input; Va_L input; t input; rs input
  function [x_L, y_L, z_L, course_L, z_L_dot, course_L_dot] = trajectory_generation(r,l,Va_L, t, rs)
    t1 = t -3*rs;
    climbing_rate = -2; % 3D
    Va_Lp = sqrt(Va_L^2-climbing_rate^2);
    omega = Va_Lp/r; % rad/s
    x_L = -l/2+r*sin(omega*t);
    y_L = l/2+r*cos(omega*t);
    z_L = -90+climbing_rate*t1; % 3D
    % z_L = -90+10*sin(3*omega*t); % 3D
    % z_L = -90; %2D
    
    x_L_dot = r*omega*cos(omega*t);
    y_L_dot = -r*omega*sin(omega*t);
    z_L_dot = climbing_rate; % 3D
    % z_L_dot = 30*cos(3*omega*t); % 3D
    % z_L_dot = 0; % 2D

    x_L_dotdot = -r*omega^2*sin(omega*t);
    y_L_dotdot = -r*omega^2*cos(omega*t);
    course_L = atan2(y_L_dot,x_L_dot);
    course_L_dot = (y_L_dotdot*x_L_dot-x_L_dotdot*y_L_dot)/(x_L_dot^2+y_L_dot^2);
end

== matlab function FW_formation_control_wind/Virtual Leader Trajectory/Mixed trajectory(NED)/Switch Case Action Subsystem6/Line trajectory(NED) ==
  data: x_L output; y_L output; z_L output; course_L output; z_L_dot output; course_L_dot output; Va_L input; t input; r input; l input; rs input
function [x_L, y_L, z_L, course_L, z_L_dot, course_L_dot] = trajectory_generation(Va_L, t,r,l, rs)
    climbing_rate = 0; % 3D
    Va_Lp = sqrt(Va_L^2-climbing_rate^2);
    x_L = -l/2+Va_Lp*t*sin(pi/2);    
    y_L = l/2+r;
    % z_L = -90;
    z_L = -90-2*rs; % 3D

    x_L_dot = Va_Lp*sin(pi/2);
    y_L_dot = 0;
    % z_L_dot = 0;
    z_L_dot = climbing_rate; % 3D
    course_L = atan2(y_L_dot,x_L_dot);
    course_L_dot = 0;
end

== matlab function FW_formation_control_wind/Virtual Leader Trajectory/Mixed trajectory(NED)/Switch Case Action Subsystem7/Circle trajectory(NED) ==
  data: x_L output; y_L output; z_L output; course_L output; z_L_dot output; course_L_dot output; r input; l input; Va_L input; t input; rs input
  function [x_L, y_L, z_L, course_L, z_L_dot, course_L_dot] = trajectory_generation(r,l,Va_L, t, rs)
    t1 = t - 0*rs;
    climbing_rate = 2; % 3D descent
    Va_Lp = sqrt(Va_L^2-climbing_rate^2);
    omega = Va_Lp/r; % rad/s
    x_L = l/2+r*sin(omega*t);
    y_L = l/2+r*cos(omega*t);
    z_L = -90-2*rs+climbing_rate*t1; % 3D
    % z_L = -90+10*sin(3*omega*t); % 3D
    % z_L = -90; %2D
    
    x_L_dot = r*omega*cos(omega*t);
    y_L_dot = -r*omega*sin(omega*t);
    z_L_dot = climbing_rate; % 3D
    % z_L_dot = 30*cos(3*omega*t); % 3D
    % z_L_dot = 0; % 2D

    x_L_dotdot = -r*omega^2*sin(omega*t);
    y_L_dotdot = -r*omega^2*cos(omega*t);
    course_L = atan2(y_L_dot,x_L_dot);
    course_L_dot = (y_L_dotdot*x_L_dot-x_L_dotdot*y_L_dot)/(x_L_dot^2+y_L_dot^2);
end

== matlab function FW_formation_control_wind/Virtual Leader Trajectory/Mixed trajectory(NED)/Switch Case Action Subsystem/Line trajectory(NED) ==
  data: x_L output; y_L output; z_L output; course_L output; z_L_dot output; course_L_dot output; Va_L input; t input; r input; l input
function [x_L, y_L, z_L, course_L, z_L_dot, course_L_dot] = trajectory_generation(Va_L, t,r,l)
    climbing_rate = 0; % 3D
    Va_Lp = sqrt(Va_L^2-climbing_rate^2);
    x_L = l/2+r;    
    y_L = l/2+Va_Lp*t*cos(-pi);
    % z_L = -90;
    z_L = -90+climbing_rate*t; % 3D
    x_L_dot = 0;
    y_L_dot = Va_Lp*cos(-pi);
    % z_L_dot = 0;
    z_L_dot = climbing_rate; % 3D
    course_L = atan2(y_L_dot,x_L_dot);
    course_L_dot = 0;
end

== matlab function FW_formation_control_wind/Virtual Leader Trajectory/Mixed trajectory(NED)/MATLAB Function ==
  data: VL input; r input; rs output; l input; ls output
function [rs,ls] = fcn(VL,r,l)
    rs = r*2*pi/VL/4;
    ls = l/VL;
end

== matlab function FW_formation_control_wind/Virtual Leader Trajectory/Mixed trajectory(NED)/MATLAB Function1 ==
  data: rs input; ls input; offset output
function offset = fcn(rs,ls)
    offset = -ls+rs;
end

== matlab function FW_formation_control_wind/Virtual Leader Trajectory/Mixed trajectory(NED)/MATLAB Function2 ==
  data: rs input; ls input; offset output
function offset = fcn(rs,ls)
    offset = -ls-rs;
end

== matlab function FW_formation_control_wind/Virtual Leader Trajectory/Mixed trajectory(NED)/MATLAB Function3 ==
  data: rs input; ls input; offset output
function offset = fcn(rs,ls)
    offset = -2*ls+rs;
end

== matlab function FW_formation_control_wind/Virtual Leader Trajectory/Mixed trajectory(NED)/MATLAB Function4 ==
  data: rs input; ls input; offset output
function offset = fcn(rs,ls)
    offset = -2*ls-2*rs;
end

== matlab function FW_formation_control_wind/Virtual Leader Trajectory/Mixed trajectory(NED)/MATLAB Function5 ==
  data: rs input; ls input; offset output
function offset = fcn(rs,ls)
    offset = -3*ls+rs;
end

== matlab function FW_formation_control_wind/Virtual Leader Trajectory/Mixed trajectory(NED)/MATLAB Function6 ==
  data: rs input; ls input; offset output
function offset = fcn(rs,ls)
    offset = -3*ls-3*rs;
end

== matlab function FW_formation_control_wind/Virtual Leader Trajectory/Mixed trajectory(NED)/MATLAB Function7 ==
  data: rs input; ls input; offset output
function offset = fcn(rs,ls)
    offset = -4*ls-3*rs;
end

== matlab function FW_formation_control_wind/Wind observer (formation frame)/Wind jerk estimation ==
  data: L input; sigma input; w_jerk_hat output
function w_jerk_hat = jerkEstimation(L, sigma)
    lamda0 = 1.1*L;
    w_jerk_hat = -lamda0*sign(sigma); 
end

== matlab function FW_formation_control_wind/Wind observer (formation frame)/wind estimation ==
  data: L input; w_ga_hat input; sigma input; wind_accel_hat output
function wind_accel_hat = accelEstimation(L, w_ga_hat, sigma)
    lambda1 = 1.5*L^(1/2);
    wind_accel_hat = - lambda1*(abs(sigma).^(1/2).*sign(sigma))+ w_ga_hat;
end

== matlab function FW_formation_control_wind/NED -> ENU ==
  data: position_NED input; position_ENU output
function position_ENU = fcn(position_NED)
R_NED_ENU = [0 1 0;
             1 0 0;
             0 0 -1;];
position_ENU = R_NED_ENU* position_NED;
end

== matlab function FW_formation_control_wind/Wind observer (formation frame)/Position estimation ==
  data: L input; w_g_hat input; sigma input; G_error_dynamic_hat output; G_error_0 input
function G_error_dynamic_hat = velocityEstimation(L, w_g_hat, sigma, G_error_0)
    lambda1 = 1.5*L^(1/2);
    G_error_dynamic_hat = G_error_0 - lambda1*(abs(sigma).^(1/2).*sign(sigma))+ w_g_hat;
end

== matlab function FW_formation_control_wind/Virtual Leader Trajectory/Mixed trajectory(NED)/determine ==
  data: ca output; t input; rs input; ls input
function ca = case_determined(t, rs, ls)
    ca = 0;
    if t < ls
        ca = 1;
    elseif (t >= ls) & (t < ls + rs)
        ca = 2;
    elseif (t >= ls + rs) & (t < 2*ls + rs)
        ca = 3;
    elseif (t >= 2*ls + rs) & (t < 2*ls + 2*rs)
        ca = 4;
    elseif (t >= 2*ls + 2*rs) & (t < 3*ls + 2*rs)
        ca = 5;
    elseif (t >= 3*ls + 2*rs) & (t < 3*ls + 3*rs)
        ca = 6;
    elseif (t >= 3*ls + 3*rs) & (t < 4*ls + 3*rs)
        ca = 7;
    elseif (t >= 4*ls + 3*rs) & (t < 4*ls + 4*rs)
        ca = 8;
    end
end

== matlab function FW_formation_control_wind/Formation Error/Geometry error  ==
  data: G_desired input; course_L input; G_error output; position_L input; position_F input
function G_error = geometry_error_generation(G_desired, course_L, position_L, position_F)
    G_error = [sin(course_L), -cos(course_L), 0 ; cos(course_L), sin(course_L), 0 ; 0, 0, -1]*(position_L - position_F) - G_desired;
end
